simulink model "sm_PID_Tuning"  (R2019a)
settings: Solver=VariableStepAuto  StartTime=0.0  StopTime=2000  RelTol=1e-3
values from neighbouring files (symbols this model uses):
  TIME_DELAY = 2.0    (= 2)    [code_DDPG_Training.m]    (also in code_Experimental_Setup.m = 2.5; code_SA_TF_Estimator.m = 2.5)
undefined symbols (not defined in the file or in its folder): sigbuilder_block
libraries: simulink x1
settings Model: Creator=rajeshs  LastModifiedBy=rajeshs

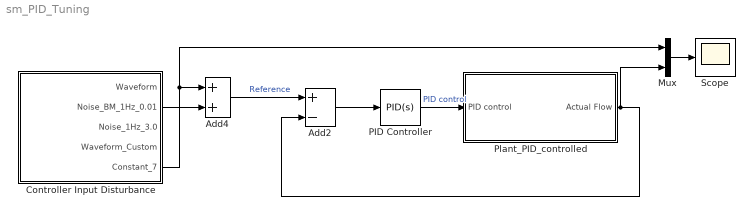
== system sm_PID_Tuning ==
  Add2 : Sum  Inputs=+-
  Add4 : Sum
  Controller Input Disturbance : Subsystem  Tag=STV Subsys  LoadFcn=sigbuilder_block('load');  StartFcn=sigbuilder_block('start');  StopFcn=sigbuilder_block('stop');  ClipboardFcn=sigbuilder_block('clipboard');  mask(Sigbuilder block){tuvar=[0:10]}
      mask help: Simulink:masks:SigbuilderBlock_MD
      mask init:
      | if ~strcmp(get_param(bdroot(gcbh),'SimulationStatus'),'stopped') tuvar = sigbuilder_block('maskInit'); end
      settings: CopyFcn=sigbuilder_block('copy');  DeleteFcn=sigbuilder_block('delete');  ModelCloseFcn=sigbuilder_block('modelClose');  PreSaveFcn=sigbuilder_block('preSave');  PauseFcn=sigbuilder_block('pause');  ContinueFcn=sigbuilder_block('continue');  NameChangeFcn=sigbuilder_block('namechange');  OpenFcn=sigbuilder_block('open',[6 63 1012.5 449.25 ]);  CloseFcn=sigbuilder_block('close');
      mask Display: plot(0, 0, 100, 100,[2, 2, 32, 32, 2], [68, 8, 8, 68, 68],[32, 2], [38, 38], [32, 19, 2],[53, 60, 44], [32, 17, 17, 2],[16, 16, 31, 31]);txt = getActiveGroup(gcbh);text(2, 100, txt,'verticalAlignment', 'top');
  Mux : Mux  Inputs=2
  PID Controller : simulink/Continuous/PID Controller  Controller=PID  Form=Parallel  TimeDomain=Continuous-time  SampleTime=-1  IntegratorMethod=Forward Euler  FilterMethod=Forward Euler  ControllerParametersSource=internal  P=0.3631  I=0.0045  D=-1.7202  UseFilter=on  N=0.0114  TunerSelectOption=Transfer Function Based (PID Tuner App)  InitialConditionSource=internal  InitialConditionForIntegrator=0  InitialConditionForFilter=0  DifferentiatorICPrevScaledInput=0  ExternalReset=none  TrackingMode=off  Kt=1  LimitOutput=off  UpperSaturationLimit=inf  LowerSaturationLimit=-inf  LinearizeAsGain=on  AntiWindupMode=none  Kb=1  POutMin=[]  POutMax=[]  IOutMin=[]  IOutMax=[]  DOutMin=[]  DOutMax=[]  NOutMin=[]  NOutMax=[]  SumOutMin=[]  SumOutMax=[]  SaturationOutMin=[]  SaturationOutMax=[]  PParamMin=[]  PParamMax=[]  IParamMin=[]  IParamMax=[]  DParamMin=[]  DParamMax=[]  NParamMin=[]  NParamMax=[]  KbParamMin=[]  KbParamMax=[]  KtParamMin=[]  KtParamMax=[]  KbOutMin=[]  KbOutMax=[]  KtOutMin=[]  KtOutMax=[]  IntegratorOutMin=[]  IntegratorOutMax=[]  FilterOutMin=[]  FilterOutMax=[]  SumI1OutMin=[]  SumI1OutMax=[]  SumI2OutMin=[]  SumI2OutMax=[]  SumI3OutMin=[]  SumI3OutMax=[]  SumI4OutMin=[]  SumI4OutMax=[]  SumDOutMin=[]  SumDOutMax=[]  DifferentiatorOutMin=[]  DifferentiatorOutMax=[]  FilterDiffOutCoefMin=[]  FilterDiffOutCoefMax=[]  ReciprocalOutMin=[]  ReciprocalOutMax=[]  SumDenOutMin=[]  SumDenOutMax=[]  SumNumOutMin=[]  SumNumOutMax=[]  DivideOutMin=[]  DivideOutMax=[]  IntegratorContinuousStateAttributes=''  IntegratorStateMustResolveToSignalObject=off  IntegratorRTWStateStorageClass=Auto  FilterContinuousStateAttributes=''  FilterStateMustResolveToSignalObject=off  FilterRTWStateStorageClass=Auto  ParallelPVariant=InternalParameters  IdealPVariant=Disabled  IVariant=InternalParameters  DVariant=InternalParameters  IntegratorVariant=Continuous  SatVariant=Disabled  AWVariant=Passthrough  PCopyVariant=Disabled  TRVariant=Disabled  FdbkBlocksVariant=Forward  IdealPFdbkVariant=Disabled  SatFdbkVariant=Disabled  DerivativeFilterVariant=ContFilter  NVariant=InternalParameters  NCopyVariant=Disabled  FilterICVariant=InternalICsFilter  IntegratorICVariant=InternalICs  ExternalResetVariant=Disabled  TRSumVariant=Passthrough  SumFdbkVariant=Disabled  SumVariant=Sum_PID
  Plant_PID_controlled : Subsystem
  Scope : Scope
  wires:
  Add2/1 -> PID Controller/1
  PID Controller/1 -> Plant_PID_controlled/1(PID control)  "PID control"
  Controller Input Disturbance/5(Constant_7) -> Mux/1, Add4/1
  Controller Input Disturbance/2(Noise_BM_1Hz_0.01) -> Add4/2
  Add4/1 -> Add2/1  "Reference"
  Plant_PID_controlled/1(Actual Flow) -> Mux/2, Add2/2
  Mux/1 -> Scope/1

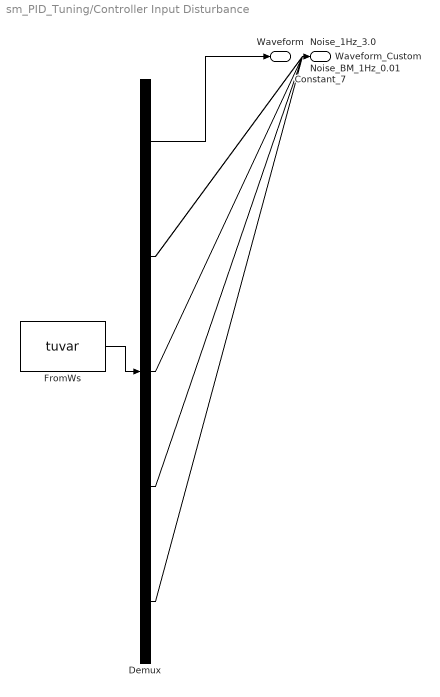
== system sm_PID_Tuning/Controller Input Disturbance ==
  Demux : Demux  Tag=STV Demux  Outputs=5
  FromWs : FromWorkspace  Tag=STV FromWs  VariableName=tuvar  SampleTime=0
      SigBuilderData=|
      | common.afterFinalStr = 'Extrapolate'
      | common.sampleTime = 0
      | dataSet.timeRange = [0 2000]
      | dataSet.name = 'Signals'
      | sbobj.Groups.Name = 'Signals'
      | sbobj.Groups.Signals(1).Name = 'Waveform'
      | sbobj.Groups.Signals(1).XData = [0 752 752 1500 1500 1750 1750 2000]
      | sbobj.Groups.Signals(1).YData = [100 100 25 25 75 75 25 25]
      | sbobj.Groups.Signals(2).Name = 'Noise_BM_1Hz_0.01'
      | sbobj.Groups.Signals(2).XData = [0 1 2 3 4 5 6 7 8 9 10 11 ... (2001 elements, 1x2001)]
      | sbobj.Groups.Signals(2).YData = [0.0109017282673 -0.00358703225346 -0.0012992763049 0.00733737523776 0.00120331570317 0.0113633128469 -0.00686773118719 0.00471682863443 0.00288342465456 0.0139185483505 -0.0134550201016 7.47406191734e-06 ... (2001 elements, 1x2001)]
      | sbobj.Groups.Signals(3).Name = 'Noise_1Hz_3.0'
      | sbobj.Groups.Signals(3).XData = [0 1 2 3 4 5 6 7 8 9 10 11 ... (2001 elements, 1x2001)]
      | sbobj.Groups.Signals(3).YData = [-1.22103016093 -2.32126408989 6.42034479721 -4.13028289214 0.366124868815 1.68201285192 -3.06458126709 -0.0302582378605 -4.3152453304 1.33545254952 0.451492702689 0.846422939597 ... (2001 elements, 1x2001)]
      | sbobj.Groups.Signals(4).Name = 'Waveform_Custom'
      | sbobj.Groups.Signals(4).XData = [0 100 110 200 290 398 500 600 1000 1050 1225 1400 1500 2000]
      | sbobj.Groups.Signals(4).YData = [75 75 100 100 100 20 20 75 75 10 10 100 100 5]
      | sbobj.Groups.Signals(5).Name = 'Constant_7'
      | sbobj.Groups.Signals(5).XData = [0 2000]
      | sbobj.Groups.Signals(5).YData = [100 100]
      | sbobj.Groups.TimeRange = [0 2000]
  Waveform : Outport  Tag=STV Outport
  Noise_BM_1Hz_0.01 : Outport  Tag=STV Outport  Port=2
  Noise_1Hz_3.0 : Outport  Tag=STV Outport  Port=3
  Waveform_Custom : Outport  Tag=STV Outport  Port=4
  Constant_7 : Outport  Tag=STV Outport  Port=5
  wires:
  Demux/1 -> Waveform/1
  FromWs/1 -> Demux/1
  Demux/2 -> Noise_BM_1Hz_0.01/1
  Demux/3 -> Noise_1Hz_3.0/1
  Demux/4 -> Waveform_Custom/1
  Demux/5 -> Constant_7/1

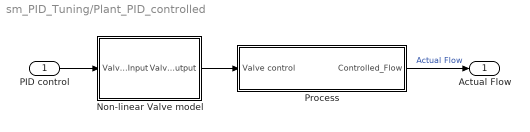
== system sm_PID_Tuning/Plant_PID_controlled ==
  PID control : Inport
  Non-linear Valve model : Subsystem
  Process : Subsystem
  Actual Flow : Outport
  wires:
  Non-linear Valve model/1(ValveOutput) -> Process/1(Valve control)
  Process/1(Controlled_Flow) -> Actual Flow/1  "Actual Flow"
  PID control/1 -> Non-linear Valve model/1(ValveInput)

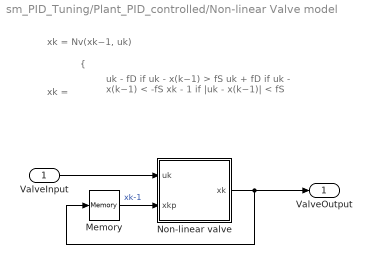
== system sm_PID_Tuning/Plant_PID_controlled/Non-linear Valve model ==
  note: xk = Nv(xk−1, uk)
  note: {
  note: xk =
  note: uk - fD if uk - x(k−1) > fS
      | uk + fD if uk - x(k−1) < -fS
      | xk - 1 if |uk - x(k−1)| < fS
  ValveInput : Inport
  Memory : Memory
  Non-linear valve : MATLAB Function  TreatAsAtomicUnit=on
  ValveOutput : Outport
  wires:
  Non-linear valve/1(xk) -> ValveOutput/1, Memory/1
  Memory/1 -> Non-linear valve/2(xkp)  "xk-1"
  ValveInput/1 -> Non-linear valve/1(uk)

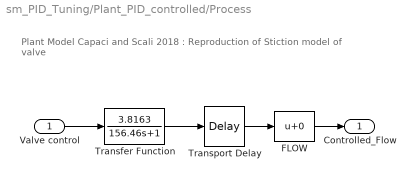
== system sm_PID_Tuning/Plant_PID_controlled/Process ==
  note: Plant Model
      |
      | Capaci and Scali 2018 : Reproduction of Stiction model of valve
  Valve control : Inport
  FLOW : Bias
  Transfer Function : TransferFcn  Numerator=[3.8163]  Denominator=[156.46 1]
  "Transport Delay " : TransportDelay  DelayTime=TIME_DELAY
  Controlled_Flow : Outport
  wires:
  FLOW/1 -> Controlled_Flow/1
  Transfer Function/1 -> "Transport Delay "/1
  Valve control/1 -> Transfer Function/1
  "Transport Delay "/1 -> FLOW/1

== matlab function sm_PID_Tuning/Plant_PID_controlled/Non-linear Valve model/Non-linear valve ==
  data: uk input; xk output; xkp input
function xk = fcn(uk, xkp)
% ----------------------------------------------------------------------------------------
% PID EVALUATION circuit Plant Model (RLVC2 | Verified 15-Jul-2020)
% Non-Linear valve model: Capaci and Scali (2018)
% Friction values conform to benchmark flow rates used in Capaci (2016)
% ----------------------------------------------------------------------------------------
% uk - fD   if uk - xk−1 > fS
% uk + fD   if uk - xk−1 < -fS
% xk - 1    if |uk - xk−1| < fS
% ----------------------------------------------------------------------------------------

    fS = 8.4;
    fD = 3.5243;
        
    t_xk = 0.0;
   
    if ((uk-xkp) > fS)
        t_xk = uk - fD;
    elseif ((uk-xkp) < -1*fS)
        t_xk = uk + fD;
    elseif (abs(uk-xkp) < fS)
        t_xk = xkp;
    end
    
xk = t_xk;
